simulink model "mconversion_nested_lib"  (Simulink 6.1)
settings: Solver=ode3  StartTime=0.0  StopTime=10.0  RelTol=1e-3
libraries: mylib x1
settings Model: Creator=awarlock  LastModifiedBy=mshakeri  ExtModeAutoUpdateStatusClock=off
settings OptimizationCC: InlineParams=on
settings DebuggingCC: CheckExecutionContextPreStartOutputMsg=on  CheckExecutionContextRuntimeOutputMsg=on

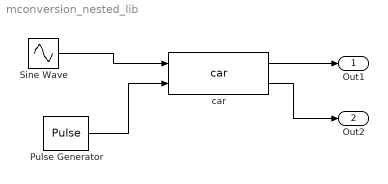
== system mconversion_nested_lib ==
  Pulse Generator : DiscretePulseGenerator  PulseType=Time based  PulseWidth=50
  Sine Wave : Sin  SampleTime=0
  car : mylib/car
  Out1 : Outport
  Out2 : Outport  Port=2
  wires:
  Sine Wave/1 -> car/1
  Pulse Generator/1 -> car/2
  car/1 -> Out1/1
  car/2 -> Out2/1
